simulink model "sysgenPolyphaseFIR"  (Simulink 7.3)
settings: Solver=ode45  StartTime=0.0  StopTime=700  RelTol=1e-3
PreLoadFcn:
  | xlrequire('PreLoadFcn')
undefined symbols (not defined in the file or in its folder): sysgenPolyphaseFIRCoeffs
libraries: xbsIndex_r4 x57, xbsCopyrightNotice_r4 x1
settings Model: Creator=alexc  LastModifiedBy=douangp
settings DataIOCC: SignalLoggingName=sigsOut
settings OptimizationCC: BlockReduction=off  BooleanDataType=off  InlineInvariantSignals=on  InitFltsAndDblsToZero=on
settings DebuggingCC: SaveWithParameterizedLinksMsg=none  SignalResolutionControl=TryResolveAllWithWarning  SolverPrmCheckMsg=none  MultiTaskDSMMsg=warning  MultiTaskCondExecSysMsg=none  StrictBusMsg=None
settings HardwareCC: TargetUnknown=on
settings RTWCC: IncludeERTFirstTime=on
settings GRTTargetCC: TargetFcnLib=ansi_tfl_tmw.mat

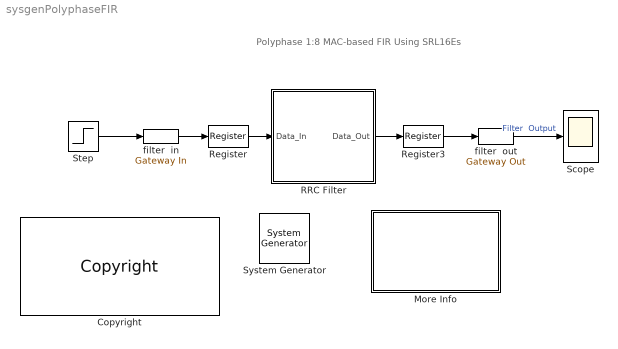
== system sysgenPolyphaseFIR ==
  note: Polyphase 1:8 MAC-based FIR Using SRL16Es
  " System Generator" : xbsIndex_r4/ System Generator  Tag=genX  SystemSampleTime=-1  xilinxfamily=virtex6  part=xc6vlx240t  speed=-1  package=ff1156  synthesis_tool=XST  clock_wrapper=Clock Enables  directory=./netlist  testbench=on  simulink_period=1  sysclk_period=4  dcm_input_clock_period=100  incr_netlist=off  trim_vbits=Everywhere in SubSystem  dbl_ovrd=According to Block Masks  core_generation=According to Block Masks  run_coregen=off  deprecated_control=off  eval_field=0  block_type=sysgen
      settings: block_version=10.1.3
  Copyright : xbsCopyrightNotice_r4/Copyright  copyrighttext="Copyright (c) 2009  by  Xilinx, Inc. All rights reserved.<br><br>This file contains proprietary, confidential information of Xilinx, Inc., is distributed under licensefrom Xilinx, Inc., and may be used, copied and/or disclosed only pursuant to the terms of a valid licenseagreement with Xilinx, Inc. Xilinx hereby grants you a license to use this file solely for design,simulation, implementation and creation of design files limited to Xilinx devices or technologies. Use with non-Xilinx devices or technologies is expressly prohibited and immediately terminates your license unless covered by a separate agreement.<br><br>Xilinx is providing this design, code, or information \"as-is\" solely for use in developing programs and solutions for Xilinx devices, with no obligation on the part of Xilinx to provide support. By providingthis design, code, or information as one possible implementation of this feature, application or standard,Xilinx is making no representation that this implementation is free from any claims of infringement. Youare responsible for obtaining any rights you may require for your implementation. Xilinx expressly disclaimsany warranty whatsoever with respect to the adequacy of the implementation, including but not limited to anywarranties or representations that this implementation is free from claims of infringement, implied warrantiesof merchantability or fitness for a particular purpose.<br><br>Xilinx products are not intended for use in life support appliances, devices, or systems. Use in such applications is expressly prohibited.<br><br>Any modifications that are made to the Source Code are done at the user's sole risk and will be unsupported.<br><br>This copyright and support notice must be retained as part of this text at all times. (c) Copyright 1995-2009 Xilinx, Inc. All rights reserved."  block_type=copyright
      settings: block_version=10.1.3
      settings: infoedit=|
      | Copyright(C) 2008 by  Xilinx, Inc. All rights reserved.<br>
      | <br>
      | This file contains proprietary, confidential information of Xilinx, Inc., is distributed under license
      | from Xilinx, Inc., and may be used, copied and/or disclosed only pursuant to the terms of a valid license
      | agreement with Xilinx, Inc. Xilinx hereby grants you a license to use this file solely for design,
      | simulation, implementation and creation of design files limited to Xilinx devices or technologies. Use
      | with non-Xilinx devices or technologies is expressly prohibited and immediately terminates your license
      | unless covered by a separate agreement.<br>
      | <br>
      | Xilinx is providing this design, code, or information "as-is" solely for use in developing programs and
      | solutions for Xilinx devices, with no obligation on the part of Xilinx to provide support. By providing
      | this design, code, or information as one possible implementation of this feature, application or standard,
      | Xilinx is making no representation that this implementation is free from any claims of infringement. You
      | are responsible for obtaining any rights you may require for your implementation. Xilinx expressly disclaims
      | any warranty whatsoever with respect to the adequacy of the implementation, including but not limited to any
      | warranties or representations that this implementation is free from claims of infringement, implied warranties
      | of merchantability or fitness for a particular purpose.<br>
      | <br>
      | Xilinx products are not intended for use in life support appliances, devices, or systems. Use in such
      | applications is expressly prohibited.<br>
      | <br>
      | Any modifications that are made to the Source Code are done at the user's sole risk and will be unsupported.<br>
      | <br>
      | This copyright and support notice must be retained as part of this text at all times.
      | (c) Copyright 1995-2008 Xilinx, Inc. All rights reserved.
  More Info : Subsystem
      mask Display: disp('Double click\n for\n more information.')
  RRC Filter : Subsystem  mask{coef=sysgenPolyphaseFIRCoeffs}
      mask prompts: coef "Coefficients"
  Register : xbsIndex_r4/Register  init=0  rst=off  en=off  dbl_ovrd=off  block_type=register
      settings: xl_area=[8 16 0 0 0 0 0]  block_version=VER_STRING_GOES_HERE
  Register3 : xbsIndex_r4/Register  init=0  rst=off  en=off  dbl_ovrd=off  block_type=register
      settings: xl_area=[8 16 0 0 0 0 0]  block_version=VER_STRING_GOES_HERE
  Scope : Scope
      settings: TimeRange=10.49142857142857  YMin=-1  YMax=1
  Step : Step  Before=1  After=0  SampleTime=32
  filter  in : xbsIndex_r4/Gateway In  arith_type=Unsigned  n_bits=16  bin_pt=0  quantization="Round  (unbiased: +/- Inf)"  overflow=Saturate  period=32  dbl_ovrd=off  timing_constraint=None  locs_specified=off  LOCs={}  block_type=gatewayin
      settings: infoedit="Gateway in block.  Converts inputs of type Simulink integer, double and fixed point to  Xilinx fixed point type.<P><P>Hardware notes:  In hardware these blocks become top level input ports."  xl_area=[0 0 0 0 16 0 0]  block_version=VER_STRING_GOES_HERE
  filter  out : xbsIndex_r4/Gateway Out  hdl_port=on  timing_constraint="Data Rate;  Set 'FAST' Attribute"  locs_specified=off  LOCs={}  block_type=gatewayout
      settings: infoedit="Gateway out block.  Converts Xilinx fixed point inputs into ouputs of type Simulink integer, double, or fixed point.<P><P>Hardware notes:  In hardware these blocks become top level output ports or are discarded, depending on how they are configured."  xl_area=[0 0 0 0 16 0 0]  block_version=VER_STRING_GOES_HERE
  wires:
  Step/1 -> filter  in/1
  filter  out/1 -> Scope/1  "Filter  Output"
  filter  in/1 -> Register/1
  Register/1 -> RRC Filter/1(Data_In)
  Register3/1 -> filter  out/1
  RRC Filter/1(Data_Out) -> Register3/1

== system sysgenPolyphaseFIR/More Info ==
  note: This design shows how a 128-tap 1:8 polyphase FIR filter can be can be
      | realized efficiently inside System Generator.  Three tricks are employed
      | to make best use of hardware:
      |
      |   - Even coefficient symmetry reduces the number of MAC engines to 4;
      |   - Engines are built from SRL16E shift registers;
      |   - Dedicated DSP48 blocks are used
      |
      | The impulse response of the filter is displayed in the output scope
      | during simulation.
      |
      | The Simulink system sample period is set to 1 in the System Generator
      | token, and the sample period of the 'filter in' gateway is 32.  This means
      | a new sample is presented to the filter every 32 system clock cycles.
      | The filter interpolates 8 to 1, so a new filter output is produced every 4
      | system clock cycles.
      |
      | The registers that precede and follow the RRC Filter subsystem are
      | mapped into IOBs, and are used to obtain accurate performance numbers.
      |
      | The design occupies 360 Slice LUTs, 395 Slice LUT-Flip Flop
      | pairs and 4 dedicated multipliers of a Xilinx xc6vlx240t-1 part. The operating
      | clock frequency is approximately 260 MHz.
  note: Polyphase 1:8 MAC-based FIR Using SRL16Es

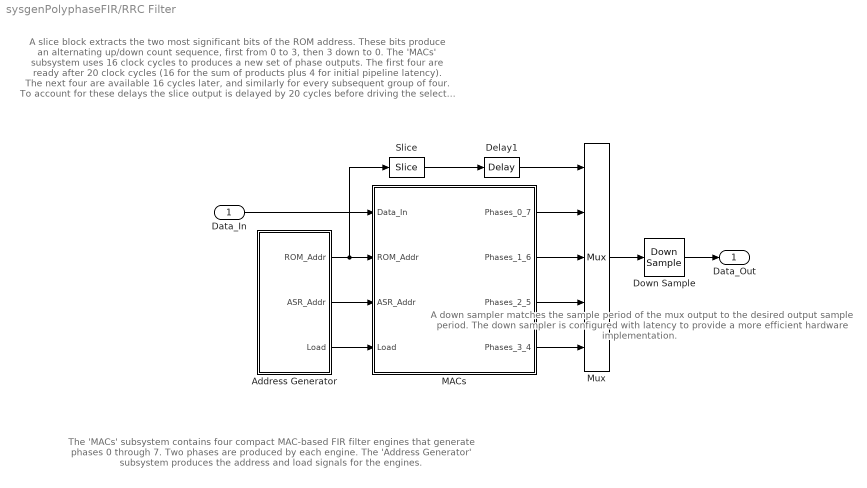
== system sysgenPolyphaseFIR/RRC Filter ==
  note: A slice block extracts the two most significant bits of the ROM address.  These
      | bits produce an alternating up/down count sequence, first from 0 to 3, then
      | 3 down to 0.   The 'MACs' subsystem uses 16 clock cycles to produces a
      | new set of phase outputs.  The first four are ready after  20 clock cycles (16 for
      | the sum of products plus 4 for initial pipeline latency).  The next four are
      | available 16 cycles later, and similarly for every subsequent group of four.
      | To account for these delays the slice output is delayed by 20 cycles before
      | driving the select line of the mux.
  note: A down sampler matches the sample
      | period of the mux output to the desired
      | output sample period. The down sampler
      | is configured with latency to provide a more
      | efficient hardware implementation.
  note: The 'MACs' subsystem contains four compact MAC-based
      | FIR filter engines that generate phases 0 through 7.  Two
      | phases are produced by each engine.  The 'Address Generator'
      | subsystem produces the address and load signals for the engines.
  Data_In : Inport  OutDataType=sfix(16)  OutScaling=2^0
  Address Generator : Subsystem
  Delay1 : xbsIndex_r4/Delay  en=off  latency=20  dbl_ovrd=off  reg_retiming=off  block_type=delay
      settings: infoedit="Delay line having  configurable length.<P><P>Hardware notes: A delay line is a chain, each link of which is an SRL16 followed by a flip-flop. If register retiming is enabled, the delay line is a chain of flip-flops."  xl_area=[2 4 0 4 0 0 0]  block_version=VER_STRING_GOES_HERE
  Down Sample : xbsIndex_r4/Down Sample  sample_ratio=4  sample_phase="Last Value of Frame  (most efficient)"  en=off  latency=1  dbl_ovrd=off  block_type=dsamp
      settings: xl_area=[8 16 0 0 0 0 0]  block_version=VER_STRING_GOES_HERE
  MACs : Subsystem
  Mux : xbsIndex_r4/Mux  inputs=4  en=off  latency=0  precision=Full  arith_type="Signed  (2's comp)"  n_bits=8  bin_pt=2  quantization=Truncate  overflow=Wrap  dbl_ovrd=off  block_type=mux
      settings: xl_area=[16 0 0 32 0 0 0]  block_version=VER_STRING_GOES_HERE
  Slice : xbsIndex_r4/Slice  nbits=2  boolean_output=off  mode=Upper Bit Location + Width  bit1=0  base1=MSB of Input  bit0=2  base0=LSB of Input  dbl_ovrd=off  block_type=slice
      settings: infoedit="Extracts a given range of bits from each input sample and presents it at the output.  The output type is ordinarily unsigned with binary point at zero, but can be Boolean when the slice is one bit wide.<P><P>Hardware notes: In hardware this block costs nothing."  block_version=VER_STRING_GOES_HERE
  Data_Out : Outport  OutDataType=sfix(16)  OutScaling=2^0
  wires:
  Address Generator/1(ROM_Addr) -> MACs/2(ROM_Addr), Slice/1
  Address Generator/2(ASR_Addr) -> MACs/3(ASR_Addr)
  Address Generator/3(Load) -> MACs/4(Load)
  MACs/4(Phases_3_4) -> Mux/5
  MACs/3(Phases_2_5) -> Mux/4
  MACs/2(Phases_1_6) -> Mux/3
  MACs/1(Phases_0_7) -> Mux/2
  Data_In/1 -> MACs/1(Data_In)
  Mux/1 -> Down Sample/1
  Slice/1 -> Delay1/1
  Delay1/1 -> Mux/1
  Down Sample/1 -> Data_Out/1

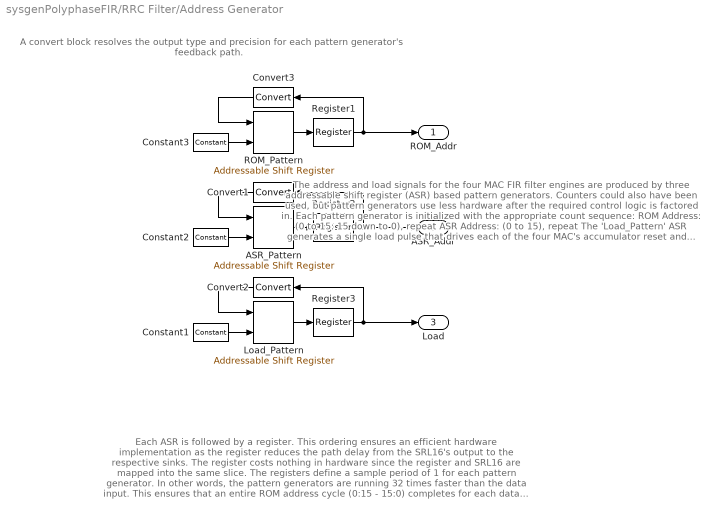
== system sysgenPolyphaseFIR/RRC Filter/Address Generator ==
  note: The address and load signals for the four MAC FIR filter engines are
      | produced by three addressable shift register (ASR) based pattern
      | generators.   Counters could also have been used, but pattern
      | generators use less hardware after the required control logic is
      | factored in.  Each pattern generator is initialized with the appropriate
      | count sequence:
      |
      | ROM Address: (0 to 15: 15 down to 0), repeat
      | ASR Address:  (0 to 15), repeat
      |
      | The 'Load_Pattern' ASR generates a single load pulse that drives
      | each of the four MAC's accumulator reset and capture register
      | enable ports.  Note the initial '1' in the ASR is not the initial output, as
      | the MAC has latency  that has been accounted for in the pattern.
  note: Each ASR is followed by a register.  This ordering ensures an
      | efficient hardware implementation as the register reduces the path
      | delay from the SRL16's output to the respective sinks.  The register
      | costs nothing in hardware since the register and SRL16 are mapped
      | into the same slice.
      |
      | The registers define a sample period of 1 for each pattern
      | generator.  In other words, the pattern generators are running
      | 32 times faster than the data input.  This ensures that an entire
      | ROM address cycle (0:15 - 15:0) completes for each data value.
      | It also defines an oversampling rate of 32 for each MAC filter engine's
      | ASR block.
  note: A convert block resolves the output type and precision
      | for each pattern generator's feedback path.
  ASR_Pattern : xbsIndex_r4/Addressable Shift Register  infer_latency=off  depth=16  initVector=fliplr(1:15)  en=off  dbl_ovrd=off  use_behavioral_HDL=off  use_rpm=off  block_type=addrsr
      settings: infoedit="Delay of configurable length.  Any element in the delay line can be addressed and driven onto the output port.<P><P>Hardware notes: Implemented using SRL16s.  If a Virtex-II device is used, multiple SRLC16s are cascaded together."  xl_area=[2 0 0 4 0 0 0]  block_version=VER_STRING_GOES_HERE
  Constant1 : xbsIndex_r4/Constant  arith_type=Unsigned  const=14  n_bits=4  bin_pt=0  explicit_period=on  period=1  equ=P=C  opselect=C  inp2=PCIN>>17  opr=+  inp1=P  carry=CIN  dbl_ovrd=off  block_type=constant
      settings: block_version=VER_STRING_GOES_HERE
  Constant2 : xbsIndex_r4/Constant  arith_type=Unsigned  const=14  n_bits=4  bin_pt=0  explicit_period=on  period=1  equ=P=C  opselect=C  inp2=PCIN>>17  opr=+  inp1=P  carry=CIN  dbl_ovrd=off  block_type=constant
      settings: block_version=VER_STRING_GOES_HERE
  Constant3 : xbsIndex_r4/Constant  arith_type=Unsigned  const=30  n_bits=5  bin_pt=0  explicit_period=on  period=1  equ=P=C  opselect=C  inp2=PCIN>>17  opr=+  inp1=P  carry=CIN  dbl_ovrd=off  block_type=constant
      settings: block_version=VER_STRING_GOES_HERE
  Convert1 : xbsIndex_r4/Convert  arith_type=Unsigned  n_bits=4  bin_pt=0  quantization=Truncate  overflow=Wrap  latency=0  dbl_ovrd=off  pipeline=off  block_type=convert
      settings: infoedit=The input is presented at the output after quantization and overflow effects.<P><P>Hardware notes: Additional hardware is used when rounding or saturation is selected and output width is less than the input width.  xl_area=[0 0 0 0 0 0 0]  block_version=VER_STRING_GOES_HERE
  Convert2 : xbsIndex_r4/Convert  arith_type=Boolean  n_bits=1  bin_pt=0  quantization=Truncate  overflow=Wrap  latency=0  dbl_ovrd=off  pipeline=off  block_type=convert
      settings: infoedit=The input is presented at the output after quantization and overflow effects.<P><P>Hardware notes: Additional hardware is used when rounding or saturation is selected and output width is less than the input width.  xl_area=[0 0 0 0 0 0 0]  block_version=VER_STRING_GOES_HERE
  Convert3 : xbsIndex_r4/Convert  arith_type=Unsigned  n_bits=4  bin_pt=0  quantization=Truncate  overflow=Wrap  latency=0  dbl_ovrd=off  pipeline=off  block_type=convert
      settings: infoedit=The input is presented at the output after quantization and overflow effects.<P><P>Hardware notes: Additional hardware is used when rounding or saturation is selected and output width is less than the input width.  xl_area=[0 0 0 0 0 0 0]  block_version=VER_STRING_GOES_HERE
  Load_Pattern : xbsIndex_r4/Addressable Shift Register  infer_latency=off  depth=16  initVector=[zeros(1,13) 1 0]  en=off  dbl_ovrd=off  use_behavioral_HDL=off  use_rpm=off  block_type=addrsr
      settings: infoedit="Delay of configurable length.  Any element in the delay line can be addressed and driven onto the output port.<P><P>Hardware notes: Implemented using SRL16s.  If a Virtex-II device is used, multiple SRLC16s are cascaded together."  xl_area=[1 0 0 1 0 0 0]  block_version=VER_STRING_GOES_HERE
  ROM_Pattern : xbsIndex_r4/Addressable Shift Register  infer_latency=off  depth=32  initVector=[(0:15) fliplr(1:15)]  en=off  dbl_ovrd=off  use_behavioral_HDL=off  use_rpm=off  block_type=addrsr
      settings: infoedit="Delay of configurable length.  Any element in the delay line can be addressed and driven onto the output port.<P><P>Hardware notes: Implemented using SRL16s.  If a Virtex-II device is used, multiple SRLC16s are cascaded together."  xl_area=[6 0 0 12 0 0 0]  block_version=VER_STRING_GOES_HERE
  Register1 : xbsIndex_r4/Register  init=0  rst=off  en=off  dbl_ovrd=off  block_type=register
      settings: xl_area=[2 4 0 0 0 0 0]  block_version=VER_STRING_GOES_HERE
  Register2 : xbsIndex_r4/Register  init=0  rst=off  en=off  dbl_ovrd=off  block_type=register
      settings: xl_area=[2 4 0 0 0 0 0]  block_version=VER_STRING_GOES_HERE
  Register3 : xbsIndex_r4/Register  init=0  rst=off  en=off  dbl_ovrd=off  block_type=register
      settings: xl_area=[1 1 0 0 0 0 0]  block_version=VER_STRING_GOES_HERE
  ROM_Addr : Outport  OutDataType=sfix(16)  OutScaling=2^0
  ASR_Addr : Outport  Port=2  OutDataType=sfix(16)  OutScaling=2^0
  Load : Outport  Port=3  OutDataType=sfix(16)  OutScaling=2^0
  wires:
  Convert1/1 -> ASR_Pattern/1
  ASR_Pattern/1 -> Register2/1
  Constant2/1 -> ASR_Pattern/2
  Register2/1 -> Convert1/1, ASR_Addr/1
  Convert3/1 -> ROM_Pattern/1
  ROM_Pattern/1 -> Register1/1
  Constant3/1 -> ROM_Pattern/2
  Register1/1 -> Convert3/1, ROM_Addr/1
  Convert2/1 -> Load_Pattern/1
  Load_Pattern/1 -> Register3/1
  Constant1/1 -> Load_Pattern/2
  Register3/1 -> Convert2/1, Load/1

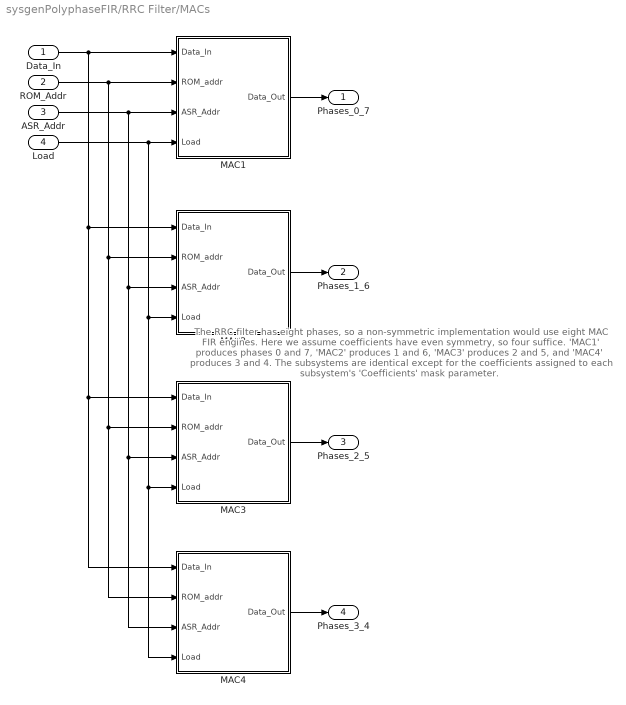
== system sysgenPolyphaseFIR/RRC Filter/MACs ==
  note: The RRC filter has eight phases, so a non-symmetric implementation
      | would use eight MAC FIR engines.  Here we assume coefficients
      | have even symmetry, so four suffice.  'MAC1' produces phases 0 and 7,
      | 'MAC2'  produces 1 and 6, 'MAC3' produces 2 and 5, and 'MAC4'
      | produces 3 and 4.  The subsystems are identical except for the
      | coefficients assigned to each subsystem's 'Coefficients' mask
      | parameter.
  Data_In : Inport  OutDataType=sfix(16)  OutScaling=2^0
  ROM_Addr : Inport  Port=2  OutDataType=sfix(16)  OutScaling=2^0
  ASR_Addr : Inport  Port=3  OutDataType=sfix(16)  OutScaling=2^0
  Load : Inport  Port=4  OutDataType=sfix(16)  OutScaling=2^0
  MAC1 : Subsystem  mask{coef=[coef(1) coef(9) coef(17) coef(25) coef(33) coef(41) coef(49) coef(57) coef(64) coef(56) coef(48) coef(40) coef(32) coef(24) coef(16) coef(8)]}
      mask prompts: coef "Coefficients"
  MAC2 : Subsystem  mask{coef=[coef(2) coef(10) coef(18) coef(26) coef(34) coef(42) coef(50) coef(58) coef(63) coef(55) coef(47) coef(39) coef(31) coef(23) coef(15) coef(7)]}
      mask prompts: coef "Coefficients"
  MAC3 : Subsystem  mask{coef=[coef(3) coef(11) coef(19) coef(27) coef(35) coef(43) coef(51) coef(59) coef(62) coef(54) coef(46) coef(38) coef(30) coef(22) coef(14) coef(6)]}
      mask prompts: coef "Coefficients"
  MAC4 : Subsystem  mask{coef=[coef(4) coef(12) coef(20) coef(28) coef(36) coef(44) coef(52) coef(60) coef(61) coef(53) coef(45) coef(37) coef(29) coef(21) coef(13) coef(5)]}
      mask prompts: coef "Coefficients"
  Phases_0_7 : Outport  OutDataType=sfix(16)  OutScaling=2^0
  Phases_1_6 : Outport  Port=2  OutDataType=sfix(16)  OutScaling=2^0
  Phases_2_5 : Outport  Port=3  OutDataType=sfix(16)  OutScaling=2^0
  Phases_3_4 : Outport  Port=4  OutDataType=sfix(16)  OutScaling=2^0
  wires:
  Data_In/1 -> MAC1/1(Data_In), MAC2/1(Data_In), MAC3/1(Data_In), MAC4/1(Data_In)
  ROM_Addr/1 -> MAC1/2(ROM_addr), MAC2/2(ROM_addr), MAC3/2(ROM_addr), MAC4/2(ROM_addr)
  MAC1/1(Data_Out) -> Phases_0_7/1
  ASR_Addr/1 -> MAC1/3(ASR_Addr), MAC2/3(ASR_Addr), MAC3/3(ASR_Addr), MAC4/3(ASR_Addr)
  Load/1 -> MAC1/4(Load), MAC3/4(Load), MAC4/4(Load), MAC2/4(Load)
  MAC3/1(Data_Out) -> Phases_2_5/1
  MAC4/1(Data_Out) -> Phases_3_4/1
  MAC2/1(Data_Out) -> Phases_1_6/1

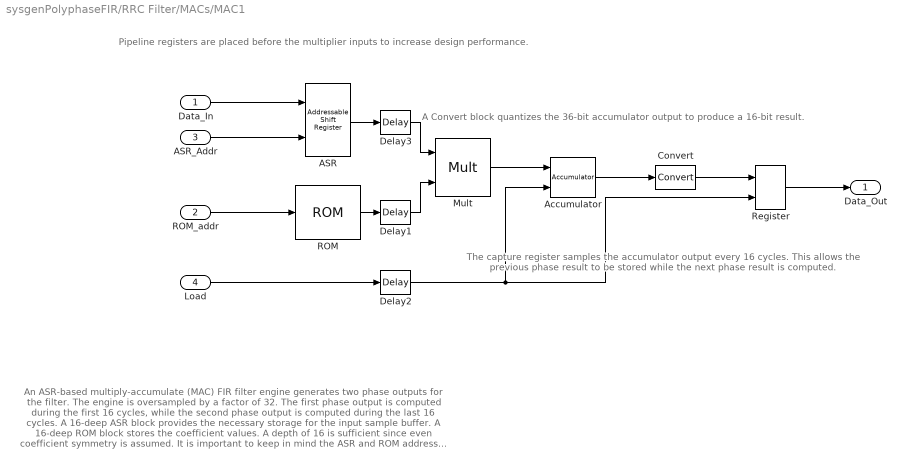
== system sysgenPolyphaseFIR/RRC Filter/MACs/MAC1 ==
  note: An ASR-based multiply-accumulate (MAC) FIR filter engine generates two phase outputs
      | for the filter.  The engine is oversampled by a factor of 32.  The first phase output is
      | computed during the first 16 cycles, while the second phase output is computed during
      | the last 16 cycles.  A 16-deep ASR block provides the necessary storage for the input
      | sample buffer.  A 16-deep ROM block stores the coefficient values.  A depth of 16 is
      | sufficient since even coefficient symmetry is assumed.  It is important to keep in mind the
      | ASR and ROM address cycles.  The ASR address is a cyclical count from 0 to 15.  The
      | ROM addresses, on the other hand, count from 0 to 15 and then from 15 down to 0.
      |
      | The MAC multiplier is configured to use the Virtex-II dedicated multipliers.  Filter
      | coefficients are stored using distributed memory, since the pipeline registers will still
      | consume extra slices if block memory were otherwise used.
  note: The capture register samples the
      | accumulator output every 16 cycles.
      | This allows the previous phase result
      | to be stored while the next phase
      | result is computed.
  note: A Convert block quantizes the 36-bit
      | accumulator output to produce a 16-bit
      | result.
  note: Pipeline registers are placed before the multiplier
      | inputs to increase design performance.
  Data_In : Inport  OutDataType=sfix(16)  OutScaling=2^0
  ROM_addr : Inport  Port=2  OutDataType=sfix(16)  OutScaling=2^0
  ASR_Addr : Inport  Port=3  OutDataType=sfix(16)  OutScaling=2^0
  Load : Inport  Port=4  OutDataType=sfix(16)  OutScaling=2^0
  ASR : xbsIndex_r4/Addressable Shift Register  infer_latency=on  depth=2  initVector=0  en=off  dbl_ovrd=off  use_behavioral_HDL=off  use_rpm=off  block_type=addrsr
      settings: infoedit="Delay of configurable length.  Any element in the delay line can be addressed and driven onto the output port.<P><P>Hardware notes: Implemented using SRL16s.  If a Virtex-II device is used, multiple SRLC16s are cascaded together."  xl_area=[8 0 0 16 0 0 0]  block_version=VER_STRING_GOES_HERE
  Accumulator : xbsIndex_r4/Accumulator  operation=Add  n_bits=36  overflow=Wrap  scale=1  rst=on  hasbypass=on  en=off  dbl_ovrd=off  use_behavioral_HDL=on  implementation=Fabric  block_type=accum
      settings: infoedit="Adder or subtractor-based accumulator.   Output type and binary point position match the input.<P><P>Hardware notes: When \"Reinitialize with Input 'b' on Reset\" is selected, the accumulator is forced to run at the system rate even if the input 'b' is running at a slower rate."  xl_area=[18 36 0 34 0 0 0]  block_version=VER_STRING_GOES_HERE
  Convert : xbsIndex_r4/Convert  arith_type="Signed  (2's comp)"  n_bits=16  bin_pt=8  quantization=Truncate  overflow=Wrap  latency=0  dbl_ovrd=off  pipeline=off  block_type=convert
      settings: infoedit=The input is presented at the output after quantization and overflow effects.<P><P>Hardware notes: Additional hardware is used when rounding or saturation is selected and output width is less than the input width.  xl_area=[0 0 0 0 0 0 0]  block_version=VER_STRING_GOES_HERE
  Delay1 : xbsIndex_r4/Delay  en=off  latency=1  dbl_ovrd=off  reg_retiming=off  block_type=delay
      settings: infoedit="Delay line having  configurable length.<P><P>Hardware notes: A delay line is a chain, each link of which is an SRL16 followed by a flip-flop. If register retiming is enabled, the delay line is a chain of flip-flops."  xl_area=[8 16 0 0 0 0 0]  block_version=VER_STRING_GOES_HERE
  Delay2 : xbsIndex_r4/Delay  en=off  latency=1  dbl_ovrd=off  reg_retiming=off  block_type=delay
      settings: infoedit="Delay line having  configurable length.<P><P>Hardware notes: A delay line is a chain, each link of which is an SRL16 followed by a flip-flop. If register retiming is enabled, the delay line is a chain of flip-flops."  xl_area=[1 1 0 0 0 0 0]  block_version=VER_STRING_GOES_HERE
  Delay3 : xbsIndex_r4/Delay  en=off  latency=1  dbl_ovrd=off  reg_retiming=off  block_type=delay
      settings: infoedit="Delay line having  configurable length.<P><P>Hardware notes: A delay line is a chain, each link of which is an SRL16 followed by a flip-flop. If register retiming is enabled, the delay line is a chain of flip-flops."  xl_area=[8 16 0 0 0 0 0]  block_version=VER_STRING_GOES_HERE
  Mult : xbsIndex_r4/Mult  precision=Full  arith_type="Signed  (2's comp)"  n_bits=20  bin_pt=12  quantization=Truncate  overflow=Wrap  en=off  latency=2  dbl_ovrd=off  use_behavioral_HDL=off  opt=Speed  use_embedded=on  optimum_pipeline=off  pipeline=on  use_rpm=off  placement_style=Rectangular shape  block_type=mult
      settings: infoedit=Multiplies two values.<P><P>Hardware notes: To use the internal pipeline stage of the dedicated multiplier you must select 'Pipeline to Greatest Extent Possible'.  xl_area=[16 32 0 0 0 1 0]  block_version=VER_STRING_GOES_HERE
  ROM : xbsIndex_r4/ROM  depth=16  initVector=coef  distributed_mem=Distributed memory  rst=off  init_reg=0  en=off  latency=0  arith_type="Signed  (2's comp)"  n_bits=16  bin_pt=15  dbl_ovrd=off  optimize=Area  use_rpm=off  block_type=sprom
      settings: xl_area=[8 0 0 16 0 0 0]  block_version=VER_STRING_GOES_HERE
  Register : xbsIndex_r4/Register  init=0  rst=off  en=on  dbl_ovrd=off  block_type=register
      settings: xl_area=[8 16 0 0 0 0 0]  block_version=VER_STRING_GOES_HERE
  Data_Out : Outport  OutDataType=sfix(16)  OutScaling=2^0
  wires:
  Data_In/1 -> ASR/1
  ROM_addr/1 -> ROM/1
  Mult/1 -> Accumulator/1
  ASR/1 -> Delay3/1
  ROM/1 -> Delay1/1
  ASR_Addr/1 -> ASR/2
  Register/1 -> Data_Out/1
  Load/1 -> Delay2/1
  Accumulator/1 -> Convert/1
  Convert/1 -> Register/1
  Delay3/1 -> Mult/1
  Delay1/1 -> Mult/2
  Delay2/1 -> Accumulator/2, Register/2

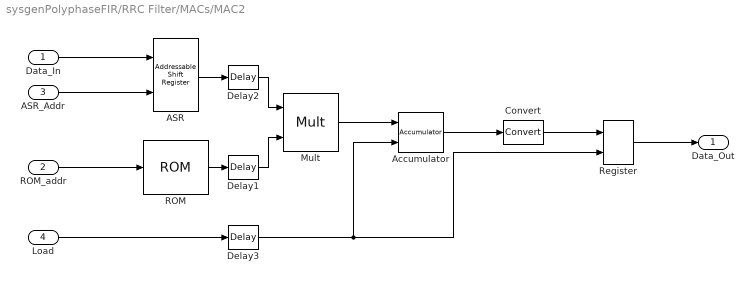
== system sysgenPolyphaseFIR/RRC Filter/MACs/MAC2 ==
  Data_In : Inport  OutDataType=sfix(16)  OutScaling=2^0
  ROM_addr : Inport  Port=2  OutDataType=sfix(16)  OutScaling=2^0
  ASR_Addr : Inport  Port=3  OutDataType=sfix(16)  OutScaling=2^0
  Load : Inport  Port=4  OutDataType=sfix(16)  OutScaling=2^0
  ASR : xbsIndex_r4/Addressable Shift Register  infer_latency=on  depth=2  initVector=0  en=off  dbl_ovrd=off  use_behavioral_HDL=off  use_rpm=off  block_type=addrsr
      settings: infoedit="Delay of configurable length.  Any element in the delay line can be addressed and driven onto the output port.<P><P>Hardware notes: Implemented using SRL16s.  If a Virtex-II device is used, multiple SRLC16s are cascaded together."  xl_area=[8 0 0 16 0 0 0]  block_version=VER_STRING_GOES_HERE
  Accumulator : xbsIndex_r4/Accumulator  operation=Add  n_bits=36  overflow=Wrap  scale=1  rst=on  hasbypass=on  en=off  dbl_ovrd=off  use_behavioral_HDL=on  implementation=Fabric  block_type=accum
      settings: infoedit="Adder or subtractor-based accumulator.   Output type and binary point position match the input.<P><P>Hardware notes: When \"Reinitialize with Input 'b' on Reset\" is selected, the accumulator is forced to run at the system rate even if the input 'b' is running at a slower rate."  xl_area=[18 36 0 34 0 0 0]  block_version=VER_STRING_GOES_HERE
  Convert : xbsIndex_r4/Convert  arith_type="Signed  (2's comp)"  n_bits=16  bin_pt=8  quantization=Truncate  overflow=Wrap  latency=0  dbl_ovrd=off  pipeline=off  block_type=convert
      settings: infoedit=The input is presented at the output after quantization and overflow effects.<P><P>Hardware notes: Additional hardware is used when rounding or saturation is selected and output width is less than the input width.  xl_area=[0 0 0 0 0 0 0]  block_version=VER_STRING_GOES_HERE
  Delay1 : xbsIndex_r4/Delay  en=off  latency=1  dbl_ovrd=off  reg_retiming=off  block_type=delay
      settings: infoedit="Delay line having  configurable length.<P><P>Hardware notes: A delay line is a chain, each link of which is an SRL16 followed by a flip-flop. If register retiming is enabled, the delay line is a chain of flip-flops."  xl_area=[8 16 0 0 0 0 0]  block_version=VER_STRING_GOES_HERE
  Delay2 : xbsIndex_r4/Delay  en=off  latency=1  dbl_ovrd=off  reg_retiming=off  block_type=delay
      settings: infoedit="Delay line having  configurable length.<P><P>Hardware notes: A delay line is a chain, each link of which is an SRL16 followed by a flip-flop. If register retiming is enabled, the delay line is a chain of flip-flops."  xl_area=[8 16 0 0 0 0 0]  block_version=VER_STRING_GOES_HERE
  Delay3 : xbsIndex_r4/Delay  en=off  latency=1  dbl_ovrd=off  reg_retiming=off  block_type=delay
      settings: infoedit="Delay line having  configurable length.<P><P>Hardware notes: A delay line is a chain, each link of which is an SRL16 followed by a flip-flop. If register retiming is enabled, the delay line is a chain of flip-flops."  xl_area=[1 1 0 0 0 0 0]  block_version=VER_STRING_GOES_HERE
  Mult : xbsIndex_r4/Mult  precision=Full  arith_type="Signed  (2's comp)"  n_bits=20  bin_pt=12  quantization=Truncate  overflow=Wrap  en=off  latency=2  dbl_ovrd=off  use_behavioral_HDL=off  opt=Speed  use_embedded=on  optimum_pipeline=off  pipeline=on  use_rpm=off  placement_style=Rectangular shape  block_type=mult
      settings: infoedit=Multiplies two values.<P><P>Hardware notes: To use the internal pipeline stage of the dedicated multiplier you must select 'Pipeline to Greatest Extent Possible'.  xl_area=[16 32 0 0 0 1 0]  block_version=VER_STRING_GOES_HERE
  ROM : xbsIndex_r4/ROM  depth=16  initVector=coef  distributed_mem=Distributed memory  rst=off  init_reg=0  en=off  latency=0  arith_type="Signed  (2's comp)"  n_bits=16  bin_pt=15  dbl_ovrd=off  optimize=Area  use_rpm=off  block_type=sprom
      settings: xl_area=[8 0 0 16 0 0 0]  block_version=VER_STRING_GOES_HERE
  Register : xbsIndex_r4/Register  init=0  rst=off  en=on  dbl_ovrd=off  block_type=register
      settings: xl_area=[8 16 0 0 0 0 0]  block_version=VER_STRING_GOES_HERE
  Data_Out : Outport  OutDataType=sfix(16)  OutScaling=2^0
  wires:
  Data_In/1 -> ASR/1
  ROM_addr/1 -> ROM/1
  Mult/1 -> Accumulator/1
  ASR/1 -> Delay2/1
  ROM/1 -> Delay1/1
  ASR_Addr/1 -> ASR/2
  Register/1 -> Data_Out/1
  Load/1 -> Delay3/1
  Accumulator/1 -> Convert/1
  Convert/1 -> Register/1
  Delay2/1 -> Mult/1
  Delay1/1 -> Mult/2
  Delay3/1 -> Accumulator/2, Register/2

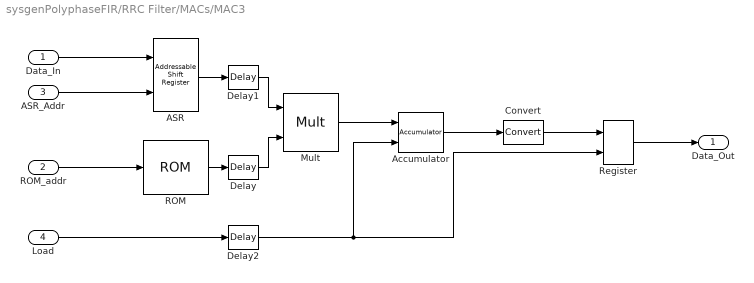
== system sysgenPolyphaseFIR/RRC Filter/MACs/MAC3 ==
  Data_In : Inport  OutDataType=sfix(16)  OutScaling=2^0
  ROM_addr : Inport  Port=2  OutDataType=sfix(16)  OutScaling=2^0
  ASR_Addr : Inport  Port=3  OutDataType=sfix(16)  OutScaling=2^0
  Load : Inport  Port=4  OutDataType=sfix(16)  OutScaling=2^0
  ASR : xbsIndex_r4/Addressable Shift Register  infer_latency=on  depth=2  initVector=0  en=off  dbl_ovrd=off  use_behavioral_HDL=off  use_rpm=off  block_type=addrsr
      settings: infoedit="Delay of configurable length.  Any element in the delay line can be addressed and driven onto the output port.<P><P>Hardware notes: Implemented using SRL16s.  If a Virtex-II device is used, multiple SRLC16s are cascaded together."  xl_area=[8 0 0 16 0 0 0]  block_version=VER_STRING_GOES_HERE
  Accumulator : xbsIndex_r4/Accumulator  operation=Add  n_bits=36  overflow=Wrap  scale=1  rst=on  hasbypass=on  en=off  dbl_ovrd=off  use_behavioral_HDL=on  implementation=Fabric  block_type=accum
      settings: infoedit="Adder or subtractor-based accumulator.   Output type and binary point position match the input.<P><P>Hardware notes: When \"Reinitialize with Input 'b' on Reset\" is selected, the accumulator is forced to run at the system rate even if the input 'b' is running at a slower rate."  xl_area=[18 36 0 34 0 0 0]  block_version=VER_STRING_GOES_HERE
  Convert : xbsIndex_r4/Convert  arith_type="Signed  (2's comp)"  n_bits=16  bin_pt=8  quantization=Truncate  overflow=Wrap  latency=0  dbl_ovrd=off  pipeline=off  block_type=convert
      settings: infoedit=The input is presented at the output after quantization and overflow effects.<P><P>Hardware notes: Additional hardware is used when rounding or saturation is selected and output width is less than the input width.  xl_area=[0 0 0 0 0 0 0]  block_version=VER_STRING_GOES_HERE
  Delay : xbsIndex_r4/Delay  en=off  latency=1  dbl_ovrd=off  reg_retiming=off  block_type=delay
      settings: infoedit="Delay line having  configurable length.<P><P>Hardware notes: A delay line is a chain, each link of which is an SRL16 followed by a flip-flop. If register retiming is enabled, the delay line is a chain of flip-flops."  xl_area=[8 16 0 0 0 0 0]  block_version=VER_STRING_GOES_HERE
  Delay1 : xbsIndex_r4/Delay  en=off  latency=1  dbl_ovrd=off  reg_retiming=off  block_type=delay
      settings: infoedit="Delay line having  configurable length.<P><P>Hardware notes: A delay line is a chain, each link of which is an SRL16 followed by a flip-flop. If register retiming is enabled, the delay line is a chain of flip-flops."  xl_area=[8 16 0 0 0 0 0]  block_version=VER_STRING_GOES_HERE
  Delay2 : xbsIndex_r4/Delay  en=off  latency=1  dbl_ovrd=off  reg_retiming=off  block_type=delay
      settings: infoedit="Delay line having  configurable length.<P><P>Hardware notes: A delay line is a chain, each link of which is an SRL16 followed by a flip-flop. If register retiming is enabled, the delay line is a chain of flip-flops."  xl_area=[1 1 0 0 0 0 0]  block_version=VER_STRING_GOES_HERE
  Mult : xbsIndex_r4/Mult  precision=Full  arith_type="Signed  (2's comp)"  n_bits=20  bin_pt=12  quantization=Truncate  overflow=Wrap  en=off  latency=2  dbl_ovrd=off  use_behavioral_HDL=off  opt=Speed  use_embedded=on  optimum_pipeline=off  pipeline=on  use_rpm=off  placement_style=Rectangular shape  block_type=mult
      settings: infoedit=Multiplies two values.<P><P>Hardware notes: To use the internal pipeline stage of the dedicated multiplier you must select 'Pipeline to Greatest Extent Possible'.  xl_area=[16 32 0 0 0 1 0]  block_version=VER_STRING_GOES_HERE
  ROM : xbsIndex_r4/ROM  depth=16  initVector=coef  distributed_mem=Distributed memory  rst=off  init_reg=0  en=off  latency=0  arith_type="Signed  (2's comp)"  n_bits=16  bin_pt=15  dbl_ovrd=off  optimize=Area  use_rpm=off  block_type=sprom
      settings: xl_area=[8 0 0 16 0 0 0]  block_version=VER_STRING_GOES_HERE
  Register : xbsIndex_r4/Register  init=0  rst=off  en=on  dbl_ovrd=off  block_type=register
      settings: xl_area=[8 16 0 0 0 0 0]  block_version=VER_STRING_GOES_HERE
  Data_Out : Outport  OutDataType=sfix(16)  OutScaling=2^0
  wires:
  Data_In/1 -> ASR/1
  ROM_addr/1 -> ROM/1
  Mult/1 -> Accumulator/1
  ASR/1 -> Delay1/1
  ROM/1 -> Delay/1
  ASR_Addr/1 -> ASR/2
  Register/1 -> Data_Out/1
  Load/1 -> Delay2/1
  Accumulator/1 -> Convert/1
  Convert/1 -> Register/1
  Delay1/1 -> Mult/1
  Delay/1 -> Mult/2
  Delay2/1 -> Accumulator/2, Register/2

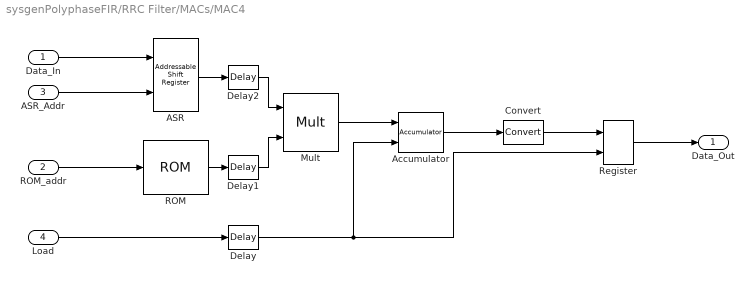
== system sysgenPolyphaseFIR/RRC Filter/MACs/MAC4 ==
  Data_In : Inport  OutDataType=sfix(16)  OutScaling=2^0
  ROM_addr : Inport  Port=2  OutDataType=sfix(16)  OutScaling=2^0
  ASR_Addr : Inport  Port=3  OutDataType=sfix(16)  OutScaling=2^0
  Load : Inport  Port=4  OutDataType=sfix(16)  OutScaling=2^0
  ASR : xbsIndex_r4/Addressable Shift Register  infer_latency=on  depth=2  initVector=0  en=off  dbl_ovrd=off  use_behavioral_HDL=off  use_rpm=off  block_type=addrsr
      settings: infoedit="Delay of configurable length.  Any element in the delay line can be addressed and driven onto the output port.<P><P>Hardware notes: Implemented using SRL16s.  If a Virtex-II device is used, multiple SRLC16s are cascaded together."  xl_area=[8 0 0 16 0 0 0]  block_version=VER_STRING_GOES_HERE
  Accumulator : xbsIndex_r4/Accumulator  operation=Add  n_bits=36  overflow=Wrap  scale=1  rst=on  hasbypass=on  en=off  dbl_ovrd=off  use_behavioral_HDL=on  implementation=Fabric  block_type=accum
      settings: infoedit="Adder or subtractor-based accumulator.   Output type and binary point position match the input.<P><P>Hardware notes: When \"Reinitialize with Input 'b' on Reset\" is selected, the accumulator is forced to run at the system rate even if the input 'b' is running at a slower rate."  xl_area=[18 36 0 34 0 0 0]  block_version=VER_STRING_GOES_HERE
  Convert : xbsIndex_r4/Convert  arith_type="Signed  (2's comp)"  n_bits=16  bin_pt=8  quantization=Truncate  overflow=Wrap  latency=0  dbl_ovrd=off  pipeline=off  block_type=convert
      settings: infoedit=The input is presented at the output after quantization and overflow effects.<P><P>Hardware notes: Additional hardware is used when rounding or saturation is selected and output width is less than the input width.  xl_area=[0 0 0 0 0 0 0]  block_version=VER_STRING_GOES_HERE
  Delay : xbsIndex_r4/Delay  en=off  latency=1  dbl_ovrd=off  reg_retiming=off  block_type=delay
      settings: infoedit="Delay line having  configurable length.<P><P>Hardware notes: A delay line is a chain, each link of which is an SRL16 followed by a flip-flop. If register retiming is enabled, the delay line is a chain of flip-flops."  xl_area=[1 1 0 0 0 0 0]  block_version=VER_STRING_GOES_HERE
  Delay1 : xbsIndex_r4/Delay  en=off  latency=1  dbl_ovrd=off  reg_retiming=off  block_type=delay
      settings: infoedit="Delay line having  configurable length.<P><P>Hardware notes: A delay line is a chain, each link of which is an SRL16 followed by a flip-flop. If register retiming is enabled, the delay line is a chain of flip-flops."  xl_area=[8 16 0 0 0 0 0]  block_version=VER_STRING_GOES_HERE
  Delay2 : xbsIndex_r4/Delay  en=off  latency=1  dbl_ovrd=off  reg_retiming=off  block_type=delay
      settings: infoedit="Delay line having  configurable length.<P><P>Hardware notes: A delay line is a chain, each link of which is an SRL16 followed by a flip-flop. If register retiming is enabled, the delay line is a chain of flip-flops."  xl_area=[8 16 0 0 0 0 0]  block_version=VER_STRING_GOES_HERE
  Mult : xbsIndex_r4/Mult  precision=Full  arith_type="Signed  (2's comp)"  n_bits=20  bin_pt=12  quantization=Truncate  overflow=Wrap  en=off  latency=2  dbl_ovrd=off  use_behavioral_HDL=off  opt=Speed  use_embedded=on  optimum_pipeline=off  pipeline=on  use_rpm=off  placement_style=Rectangular shape  block_type=mult
      settings: infoedit=Multiplies two values.<P><P>Hardware notes: To use the internal pipeline stage of the dedicated multiplier you must select 'Pipeline to Greatest Extent Possible'.  xl_area=[16 32 0 0 0 1 0]  block_version=VER_STRING_GOES_HERE
  ROM : xbsIndex_r4/ROM  depth=16  initVector=coef  distributed_mem=Distributed memory  rst=off  init_reg=0  en=off  latency=0  arith_type="Signed  (2's comp)"  n_bits=16  bin_pt=15  dbl_ovrd=off  optimize=Area  use_rpm=off  block_type=sprom
      settings: xl_area=[8 0 0 16 0 0 0]  block_version=VER_STRING_GOES_HERE
  Register : xbsIndex_r4/Register  init=0  rst=off  en=on  dbl_ovrd=off  block_type=register
      settings: xl_area=[8 16 0 0 0 0 0]  block_version=VER_STRING_GOES_HERE
  Data_Out : Outport  OutDataType=sfix(16)  OutScaling=2^0
  wires:
  Data_In/1 -> ASR/1
  ROM_addr/1 -> ROM/1
  Mult/1 -> Accumulator/1
  ASR/1 -> Delay2/1
  ROM/1 -> Delay1/1
  ASR_Addr/1 -> ASR/2
  Register/1 -> Data_Out/1
  Load/1 -> Delay/1
  Accumulator/1 -> Convert/1
  Convert/1 -> Register/1
  Delay2/1 -> Mult/1
  Delay1/1 -> Mult/2
  Delay/1 -> Accumulator/2, Register/2
